simulink model "carnew"  (R2023b)
settings: Solver=ode23s  StartTime=0.0  StopTime=10.0  RelTol=1e-3
undefined symbols (not defined in the file): Ion, Lithium
libraries: spsDiodeLib x4, spsIGBTDiodeLib x4, spsSeriesRLCBranchLib x4, spsVoltageMeasurementLib x3, spsCurrentMeasurementLib x2, spsMeanLib x2, spsPowerLib x2, spsACVoltageSourceLib x1, spsBatteryLib x1, spsMutualInductanceLib x1, spsUniversalBridgeLib x1, spspowerguiLib x1
settings Model: Creator=syedi  LastModifiedBy=syedi

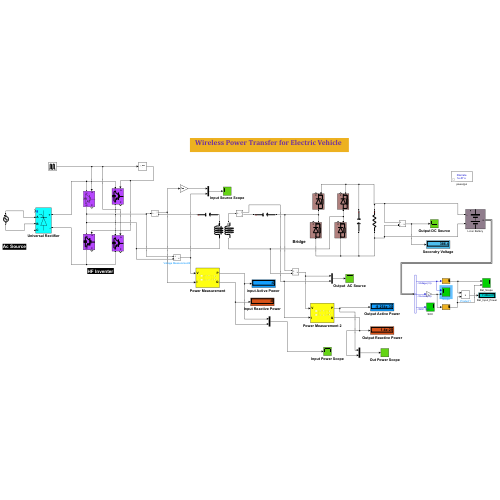
[thumbnail: Simulink's stored preview of the top-level diagram]
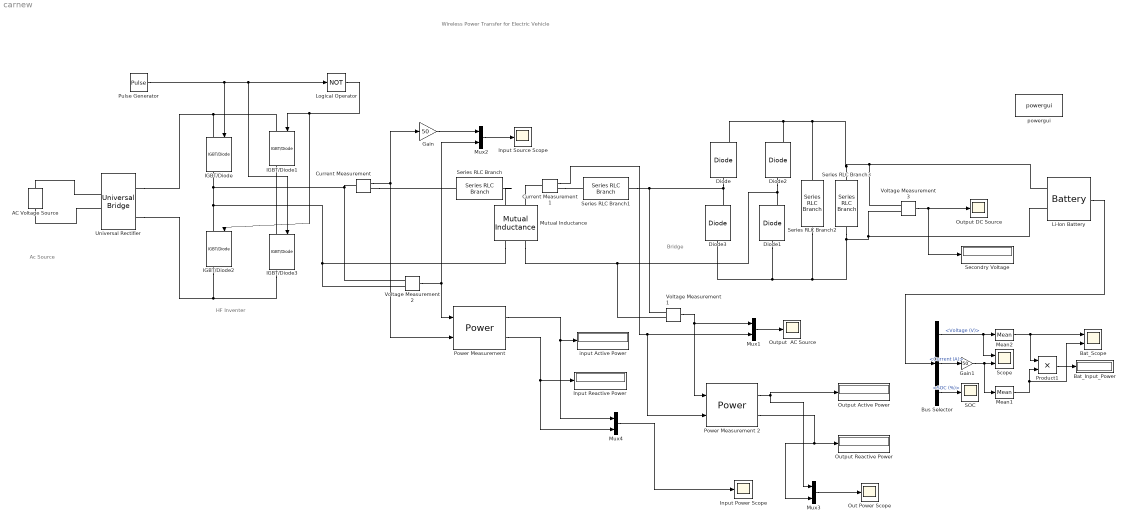
== system carnew ==
  note: Wireless Power Transfer for Electric Vehicle
  note: HF Inventer
  note: Bridge
  note: Ac Source
  AC Voltage Source : spsACVoltageSourceLib/AC Voltage Source  Amplitude=400  Phase=0  Frequency=50  SampleTime=0  Measurements=None  BusType=swing  Pref=10e3  Qref=0  Qmin=-inf  Qmax=+inf
  Bat_Input_Power : Display
  Bat_Scope : Scope  NumInputPorts=2
  Bus Selector : BusSelector  OutputSignals=Voltage (V),Current (A),SOC (%)
  Current Measurement : spsCurrentMeasurementLib/Current Measurement  PhasorSimulation=off  OutputType=Complex  PSBequivalent=0
  Current Measurement1 : spsCurrentMeasurementLib/Current Measurement  PhasorSimulation=off  OutputType=Complex  PSBequivalent=0
  Diode{,1..3} (4 alike) : spsDiodeLib/Diode  Ron=0.001  Lon=0  Vf=0.8  IC=0  UseSnubber=0  Rs=500  Cs=250e-9  Measurements=on
  Gain : Gain  Gain=50
  Gain1 : Gain  Gain=50
  IGBT/Diode{,1..3} (4 alike) : spsIGBTDiodeLib/IGBT//Diode  Ron=1e-3  Rs=1e5  Cs=inf  Measurements=on
  Input Power Scope : Scope
  Input Reactive Power : Display
  Input Source Scope : Scope
  Li-Ion Battery : spsBatteryLib/Battery  BatType=Lithium-Ion  ShowTempParam=off  ThermalPreset=no  ShowAgeParam=off  NomV=360  NomQ=100  SOC=50  Batt_Tr=10  PresetModel=on  MaxQ=100  MinV=300  FullV=465.5949  Dis_rate=43.4783  R=0.04  Normal_OP=90.4348  expZone="[432.1543      4.913043]"  current=[6.5 13 32.5]  Units=Time  Tci=20  NomT=20  T2=-30  MaxQ2=4.8  FullV2=7.1  Normal_OP2=5.655  expZone2="[6.58           1]"  Rca=0.6  ti=2000  Dp=0  Neq0=0  Tsim=1e6  Ta1=25  Qeol=5.4*0.9  Reol=0.013333*1.2  Char_age=[2.3478, 3]  Dis_age=[2.3478, 10]  N1=1500  N2=10500  N3=1000  N4=1400  Ta2=45  N5=950
  Logical Operator : Logic  Operator=NOT  AllPortsSameDT=off  OutDataTypeStr=boolean
  Mean1 : spsMeanLib/Mean  Freq=50000  Vinit=0  Ts=0
  Mean2 : spsMeanLib/Mean  Freq=50000  Vinit=0  Ts=0
  Mutual Inductance : spsMutualInductanceLib/Mutual Inductance  LConnTagsString=a|b  RConnTagsString=A|B  TypeOfMutual=Two or three windings with equal mutual terms  NumberOfWindings=3  SelfImpedance1=[.01 1e-03]  SelfImpedance2=[ .01 1e-03]  ThreeWindings=off  SelfImpedance3=[ 1.1 1.1e-03]  MutualImpedance=[.1 .1*sqrt(1e-6)]  InductanceMatrix="[1.0 0.9  0.9 ;  0.9 1.0  0.9;  0.9 0.9 1.0 ] * 1e-3"  ResistanceMatrix="[1.0 0.9  0.9 ;  0.9 1.0  0.9;  0.9 0.9 1.0 ]"  Measurements=None
      settings: LibrarySourceBlock=sps_lib/Passives/Mutual Inductance
  Mux{1..4} (4 alike) : Mux  Inputs=2
  Out Power Scope : Scope
  Output  AC Source : Scope
  Output Active Power : Display
  Output DC Source : Scope
  Output Reactive Power : Display
  Power Measurement : spsPowerLib/Power  Freq=50000  Vinit=[1, 0]  Iinit=[1, 0]  Ts=0
  Power Measurement 2 : spsPowerLib/Power  Freq=50000  Vinit=[1, 0]  Iinit=[1, 0]  Ts=0
  Product1 : Product
  Pulse Generator : DiscretePulseGenerator  PulseType=Time based  Period=1/50000  PulseWidth=50
  SOC : Scope
  Scope : Scope  NumInputPorts=2
  Secondry Voltage : Display
  Series RLC Branch : spsSeriesRLCBranchLib/Series RLC Branch  LConnTagsString=__new0  RConnTagsString=__new0  BranchType=C  Resistance=1  Inductance=1e-3  SetiL0=off  InitialCurrent=0  Capacitance=1.0132e-08  Setx0=off  InitialVoltage=0  Measurements=None
  Series RLC Branch1 : spsSeriesRLCBranchLib/Series RLC Branch  LConnTagsString=__new0  RConnTagsString=__new0  BranchType=C  Resistance=1  Inductance=1e-3  SetiL0=off  InitialCurrent=0  Capacitance=1.0132e-08  Setx0=off  InitialVoltage=0  Measurements=None
  Series RLC Branch2 : spsSeriesRLCBranchLib/Series RLC Branch  LConnTagsString=__new0  RConnTagsString=__new0  BranchType=C  Resistance=1  Inductance=1e-3  SetiL0=off  InitialCurrent=0  Capacitance=220e-6  Setx0=off  InitialVoltage=0  Measurements=None
  Series RLC Branch3 : spsSeriesRLCBranchLib/Series RLC Branch  LConnTagsString=__new0  RConnTagsString=__new0  BranchType=R  Resistance=10  Inductance=1e-3  SetiL0=off  InitialCurrent=0  Capacitance=1e-6  Setx0=off  InitialVoltage=0  Measurements=None
  Universal Rectifier : spsUniversalBridgeLib/Universal Bridge  Arms=3  SnubberResistance=1e5  SnubberCapacitance=inf  Device=Thyristors  Ron=1e-3  Lon=0  ForwardVoltages="[  0  0  ]"  ForwardVoltage=0  GTOparameters=[ 10e-6 , 20e-6 ]  IGBTparameters=[ 1e-6 , 2e-6 ]  Measurements=None  Measurements_2=None  converterType=Rectifier
  Voltage Measurement1 : spsVoltageMeasurementLib/Voltage Measurement  PhasorSimulation=off  OutputType=Complex  PSBequivalent=0
  Voltage Measurement2 : spsVoltageMeasurementLib/Voltage Measurement  PhasorSimulation=off  OutputType=Complex  PSBequivalent=0
  Voltage Measurement3 : spsVoltageMeasurementLib/Voltage Measurement  PhasorSimulation=off  OutputType=Complex  PSBequivalent=0
  "input Active Power " : Display
  powergui : spspowerguiLib/powergui  Priority=1  SimulationMode=Discrete  SampleTime=1e-7  frequency=60  Iterations=50  frequencyindice=0  Pbase=100e6  ErrMax=1e-4  UnitsV=kV  UnitsW=MW  buscounter=0  FunctionMessages=off  echomessages=off  EnableUseOfTLC=off  CurrentSourceSwitches=off  DisableSnubberDevices=off  DisableRonSwitches=off  DisableVfSwitches=off  DisplayEquations=off  AutomaticDiscreteSolvers=off  SolverType=Tustin/Backward Euler (TBE)  Interpol=off  ExternalGateDelay=off  methode=off  Ts=100  x0status=blocks  SPID=on  SwTol=0  HookPort=off  NonlinearTolerance=1e-4  nMaxIteration=100  ContinueOnMaxIteration=off  RestoreLinks=warning  ResistiveCurrentMeasurement=off  Frange=[0:2:500]  Ylog=off  Xlog=on  ShowGrid=off  save=off  variable=ZData  structure=source  ZoomFFT=off  StartTime=0.1  cycles=5  DisplayStyle=2  fundamental=50  FreqAxis=on  MaxFrequency=1000  frequencyindicesteady=1  RmsSteady=1  display=off
  wires:
  Voltage Measurement1/1 -> Power Measurement 2/1, Mux1/1
  Current Measurement1/1 -> Power Measurement 2/2, Mux1/2
  Current Measurement/1 -> Power Measurement/2, Gain/1
  Gain/1 -> Mux2/1
  Voltage Measurement2/1 -> Power Measurement/1, Mux2/2
  Mux1/1 -> Output  AC Source/1
  Mux2/1 -> Input Source Scope/1
  Voltage Measurement3/1 -> Output DC Source/1, Secondry Voltage/1
  Pulse Generator/1 -> Logical Operator/1, IGBT/Diode3/1, IGBT/Diode/1
  Logical Operator/1 -> IGBT/Diode1/1, IGBT/Diode2/1
  Power Measurement/1 -> Mux4/1, "input Active Power "/1
  Power Measurement/2 -> Mux4/2, Input Reactive Power/1
  Power Measurement 2/1 -> Mux3/1, Output Active Power/1
  Power Measurement 2/2 -> Mux3/2, Output Reactive Power/1
  Mux3/1 -> Out Power Scope/1
  Bus Selector/3 -> SOC/1  "<SOC (%)>"
  Bus Selector/2 -> Gain1/1  "<Current (A)>"
  Gain1/1 -> Mean1/1, Scope/2
  Mean1/1 -> Bat_Scope/2, Product1/2
  Bus Selector/1 -> Mean2/1, Scope/1  "<Voltage (V)>"
  Mean2/1 -> Bat_Scope/1, Product1/1
  Product1/1 -> Bat_Input_Power/1
  Li-Ion Battery/1 -> Bus Selector/1
  Mux4/1 -> Input Power Scope/1
  connections:
  Series RLC Branch/RConn1 -- Mutual Inductance/LConn1
  Series RLC Branch3/LConn1 -- Voltage Measurement3/LConn1 -- Li-Ion Battery/LConn1 -- Diode2/RConn1 -- Diode/RConn1 -- Series RLC Branch2/LConn1
  Series RLC Branch3/RConn1 -- Voltage Measurement3/LConn2 -- Li-Ion Battery/LConn2 -- Diode1/LConn1 -- Diode3/LConn1 -- Series RLC Branch2/RConn1
  Diode2/LConn1 -- Mutual Inductance/RConn2 -- Voltage Measurement1/LConn2 -- Diode1/RConn1
  Diode/LConn1 -- Series RLC Branch1/RConn1 -- Voltage Measurement1/LConn1 -- Diode3/RConn1
  IGBT/Diode1/LConn1 -- Universal Rectifier/RConn1 -- IGBT/Diode/LConn1
  IGBT/Diode2/LConn1 -- Voltage Measurement2/LConn1 -- Current Measurement/LConn1 -- IGBT/Diode/RConn1 -- Voltage Measurement2/LConn2 -- Mutual Inductance/RConn1
  IGBT/Diode3/LConn1 -- IGBT/Diode1/RConn1
  IGBT/Diode3/RConn1 -- Universal Rectifier/RConn2 -- IGBT/Diode2/RConn1
  Current Measurement/RConn1 -- Series RLC Branch/LConn1
  Current Measurement1/RConn1 -- Series RLC Branch1/LConn1
  Current Measurement1/LConn1 -- Mutual Inductance/LConn2
  AC Voltage Source/RConn1 -- Universal Rectifier/LConn1
  Universal Rectifier/LConn2 -- AC Voltage Source/LConn1
